simulink model "Day_1_Power_Electronics"  (R2021a)
settings: Solver=VariableStepAuto  StartTime=0.0  StopTime=10.0  RelTol=1e-3
settings Model: Creator=User  LastModifiedBy=User

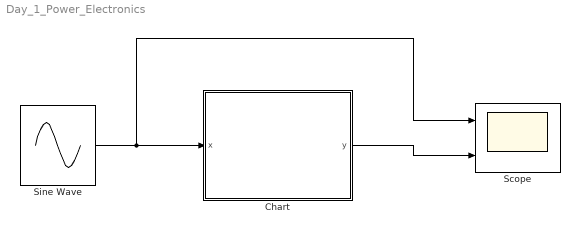
== system Day_1_Power_Electronics ==
  Chart : Stateflow chart  TreatAsAtomicUnit=on
  Scope : Scope  NumInputPorts=2
  Sine Wave : Sin  SampleTime=0.2
  wires:
  Sine Wave/1 -> Scope/1, Chart/1(x)
  Chart/1(y) -> Scope/2

== stateflow chart Day_1_Power_Electronics/Chart ==
  state On
    y=x;
  state Off
    y=0;
  (default) -> On
  On -> Off : [x<t0]
  Off -> On : [x>t0]
  data: x input; y output; t0 constant double =0
